simulink model "pid_active_suspension"  (R2024b)
settings: Solver=FixedStepAuto  StartTime=0.0  StopTime=10.0  FixedStep=0.001  MaxStep=0.001  RelTol=1e-3
undefined symbols (not defined in the file): A, B, C, D, kw, sigbuilder_block, T
libraries: slpidlib x1, simulink x1, dspfdesign x1
settings Model: Creator=11508  LastModifiedBy=11508
settings DataIOCC: SaveFormat=Array  ReturnWorkspaceOutputs=off
settings OptimizationCC: ReuseModelBlockBuffer=off
settings DebuggingCC: AlgebraicLoopMsg=none
settings RTWCC: GPUComputeCapability=3.5

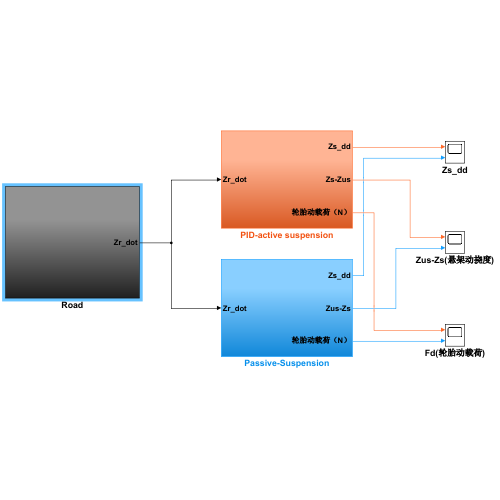
[thumbnail: Simulink's stored preview of the top-level diagram]
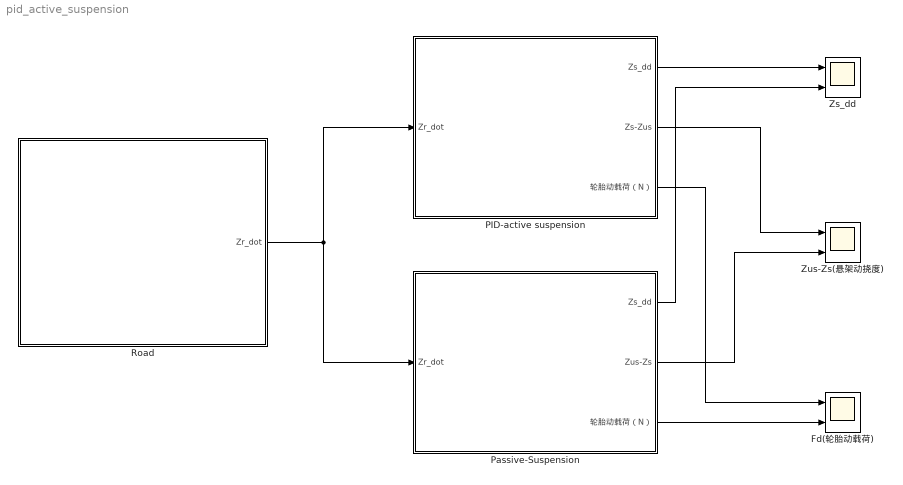
== system pid_active_suspension ==
  Fd(轮胎动载荷) : Scope  NumInputPorts=2
  PID-active suspension : Subsystem
  Passive-Suspension : Subsystem
  Road : Subsystem
  Zs_dd : Scope  NumInputPorts=2
  Zus-Zs(悬架动挠度) : Scope  NumInputPorts=2
  wires:
  PID-active suspension/1(Zs_dd) -> Zs_dd/1
  Passive-Suspension/1(Zs_dd) -> Zs_dd/2
  PID-active suspension/2(Zs-Zus) -> Zus-Zs(悬架动挠度)/1
  Passive-Suspension/2(Zus-Zs) -> Zus-Zs(悬架动挠度)/2
  Passive-Suspension/3(轮胎动载荷（N）) -> Fd(轮胎动载荷)/2
  PID-active suspension/3(轮胎动载荷（N）) -> Fd(轮胎动载荷)/1
  Road/1(Zr_dot) -> PID-active suspension/1(Zr_dot), Passive-Suspension/1(Zr_dot)

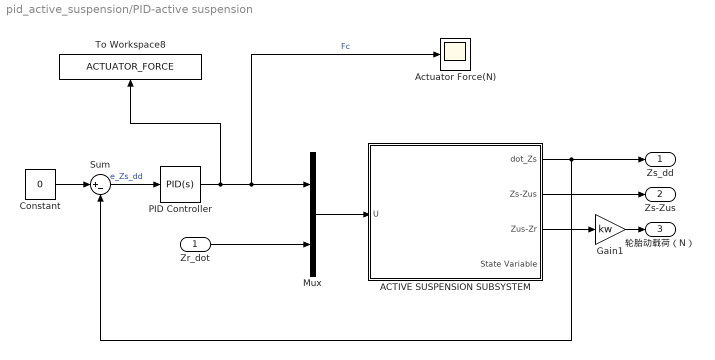
== system pid_active_suspension/PID-active suspension ==
  Zr_dot : Inport
  ACTIVE SUSPENSION SUBSYSTEM : Subsystem
  Actuator Force(N) : Scope
  Constant : Constant  Value=0
  Gain1 : Gain  Gain=kw
  Mux : Mux  Inputs=2
  PID Controller : slpidlib/PID Controller  Controller=PID  Form=Parallel  TimeDomain=Continuous-time  UseExternalTs=off  SampleTime=-1  IntegratorMethod=Forward Euler  FilterMethod=Forward Euler  ControllerParametersSource=internal  P=500  I=25  UseKiTs=off  D=10  UseExternalDerivativeSource=off  N=100  UseFilter=on  TunerSelectOption=Transfer Function Based (PID Tuner App)  InitialConditionSource=internal  InitialConditionForIntegrator=0  InitialConditionForFilter=0  DifferentiatorICPrevScaledInput=0  ExternalReset=none  TrackingMode=off  Kt=1  LimitOutput=off  SatLimitsSource=internal  UpperSaturationLimit=inf  LowerSaturationLimit=-inf  LinearizeAsGain=on  AntiWindupMode=none  Kb=1  LimitIntegrator=off  UpperIntegratorSaturationLimit=inf  LowerIntegratorSaturationLimit=-inf  POutMin=[]  POutMax=[]  IOutMin=[]  IOutMax=[]  DOutMin=[]  DOutMax=[]  NOutMin=[]  NOutMax=[]  SumOutMin=[]  SumOutMax=[]  SaturationOutMin=[]  SaturationOutMax=[]  PParamMin=[]  PParamMax=[]  IParamMin=[]  IParamMax=[]  DParamMin=[]  DParamMax=[]  NParamMin=[]  NParamMax=[]  KbParamMin=[]  KbParamMax=[]  KtParamMin=[]  KtParamMax=[]  KbOutMin=[]  KbOutMax=[]  KtOutMin=[]  KtOutMax=[]  IntegratorOutMin=[]  IntegratorOutMax=[]  FilterOutMin=[]  FilterOutMax=[]  SumI1OutMin=[]  SumI1OutMax=[]  SumI2OutMin=[]  SumI2OutMax=[]  SumI3OutMin=[]  SumI3OutMax=[]  SumI4OutMin=[]  SumI4OutMax=[]  SumDOutMin=[]  SumDOutMax=[]  DifferentiatorOutMin=[]  DifferentiatorOutMax=[]  FilterDiffOutCoefMin=[]  FilterDiffOutCoefMax=[]  ReciprocalOutMin=[]  ReciprocalOutMax=[]  SumDenOutMin=[]  SumDenOutMax=[]  SumNumOutMin=[]  SumNumOutMax=[]  DivideOutMin=[]  DivideOutMax=[]  UdiffTsProdOutMin=[]  UdiffTsProdOutMax=[]  NTsProdOutMin=[]  NTsProdOutMax=[]  UintegralTsProdOutMin=[]  UintegralTsProdOutMax=[]  UngainTsProdOutMin=[]  UngainTsProdOutMax=[]  ClampingZeroOutDataTypeStr=Inherit: Inherit via back propagation  ClampingZeroOutMin=[]  ClampingZeroOutMax=[]  FilterDenConstantOutDataTypeStr=Inherit: Inherit via back propagation  FilterDenConstantOutMin=[]  FilterDenConstantOutMax=[]  PCopyOutDataTypeStr=Inherit: Inherit via back propagation  PCopyOutMin=[]  PCopyOutMax=[]  NCopyOutDataTypeStr=Inherit: Inherit via back propagation  NCopyOutMin=[]  NCopyOutMax=[]  IntegratorContinuousStateAttributes=''  IntegratorStateMustResolveToSignalObject=off  IntegratorRTWStateStorageClass=Auto  FilterContinuousStateAttributes=''  FilterStateMustResolveToSignalObject=off  FilterRTWStateStorageClass=Auto  ParallelPVariant=InternalParameters  IdealPVariant=Disabled  IVariant=InternalParameters  DVariant=InternalParameters  IntegratorVariant=Continuous  SatVariant=Disabled  AWVariant=Passthrough  PCopyVariant=Disabled  TRVariant=Disabled  FdbkBlocksVariant=Forward  IdealPFdbkVariant=Disabled  SatFdbkVariant=Disabled  DerivativeFilterVariant=ContFilter  NVariant=InternalParameters  NCopyVariant=Disabled  FilterICVariant=InternalICsFilter  IntegratorICVariant=InternalICs  ExternalResetVariant=Disabled  TRSumVariant=Passthrough  SumFdbkVariant=Disabled  SumVariant=Sum_PID  TsampFilterVariant=InternalTs  TsampNgainVariant=Passthrough  TsampIntegralVariant=Disabled_SignalSpec  ExternalSaturationOutDataTypeStr=Inherit: Same as second input  DerivativeSourceVariant=ErrorSignal  PreIntVariant=InternalPreInt
  Sum : Sum  Inputs=|+-
  To Workspace8 : ToWorkspace  VariableName=ACTUATOR_FORCE  SampleTime=-1
  Zs_dd : Outport
  Zs-Zus : Outport  Port=2
  轮胎动载荷（N） : Outport  Port=3
  wires:
  Mux/1 -> ACTIVE SUSPENSION SUBSYSTEM/1(U)
  PID Controller/1 -> Mux/1, Actuator Force(N)/1, To Workspace8/1  "Fc"
  ACTIVE SUSPENSION SUBSYSTEM/2(Zs-Zus) -> Zs-Zus/1
  ACTIVE SUSPENSION SUBSYSTEM/3(Zus-Zr) -> Gain1/1
  Gain1/1 -> 轮胎动载荷（N）/1
  ACTIVE SUSPENSION SUBSYSTEM/1(dot_Zs) -> Sum/2, Zs_dd/1
  Zr_dot/1 -> Mux/2
  Constant/1 -> Sum/1
  Sum/1 -> PID Controller/1  "e_Zs_dd"

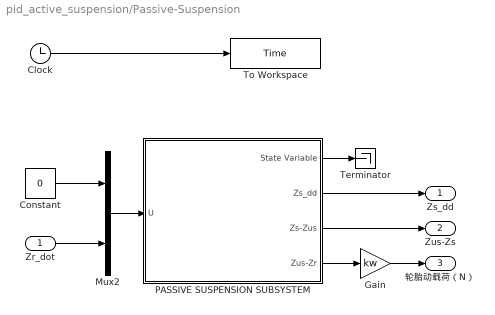
== system pid_active_suspension/Passive-Suspension ==
  Zr_dot : Inport
  Clock : Clock
  Constant : Constant  Value=0
  Gain : Gain  Gain=kw
  Mux2 : Mux  Inputs=2
  PASSIVE SUSPENSION SUBSYSTEM : Subsystem
  Terminator : Terminator
  To Workspace : ToWorkspace  VariableName=Time  SampleTime=-1
  Zs_dd : Outport
  Zus-Zs : Outport  Port=2
  轮胎动载荷（N） : Outport  Port=3
  wires:
  Mux2/1 -> PASSIVE SUSPENSION SUBSYSTEM/1(U)
  PASSIVE SUSPENSION SUBSYSTEM/3(Zs-Zus) -> Zus-Zs/1
  PASSIVE SUSPENSION SUBSYSTEM/2(Zs_dd) -> Zs_dd/1
  Gain/1 -> 轮胎动载荷（N）/1
  PASSIVE SUSPENSION SUBSYSTEM/4(Zus-Zr) -> Gain/1
  Zr_dot/1 -> Mux2/2
  Constant/1 -> Mux2/1
  Clock/1 -> To Workspace/1
  PASSIVE SUSPENSION SUBSYSTEM/1(State Variable) -> Terminator/1

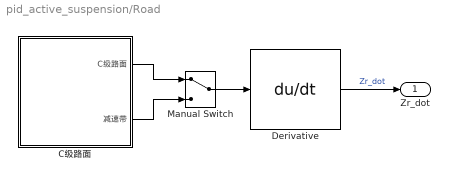
== system pid_active_suspension/Road ==
  C级路面 : Subsystem
  Derivative : Derivative
  Manual Switch : ManualSwitch
  Zr_dot : Outport
  wires:
  Derivative/1 -> Zr_dot/1  "Zr_dot"
  C级路面/2(减速带) -> Manual Switch/2
  C级路面/1(C级路面) -> Manual Switch/1
  Manual Switch/1 -> Derivative/1

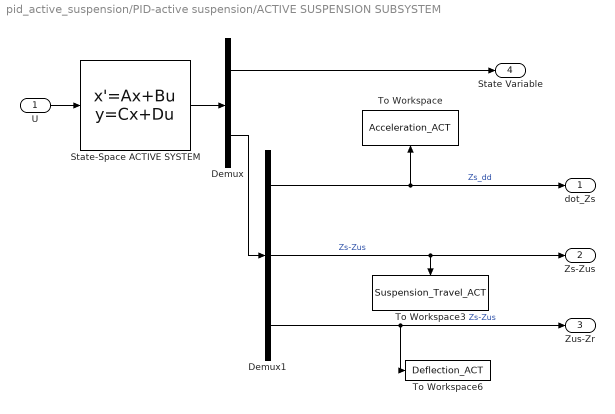
== system pid_active_suspension/PID-active suspension/ACTIVE SUSPENSION SUBSYSTEM ==
  U : Inport
  Demux : Demux  Outputs=[4 3]
  Demux1 : Demux  Outputs=3
  State-Space ACTIVE SYSTEM : StateSpace  A=A  B=cat(2,B,E)  C=cat(1,eye(4), C)  D=cat(1,zeros(4,2),cat(2,D,T))  InitialCondition=0
  To Workspace : ToWorkspace  VariableName=Acceleration_ACT  SampleTime=-1
  To Workspace3 : ToWorkspace  VariableName=Suspension_Travel_ACT  SampleTime=-1
  To Workspace6 : ToWorkspace  VariableName=Deflection_ACT  SampleTime=-1
  dot_Zs : Outport
  Zs-Zus : Outport  Port=2
  Zus-Zr : Outport  Port=3
  State Variable : Outport  Port=4
  wires:
  Demux/1 -> State Variable/1
  State-Space ACTIVE SYSTEM/1 -> Demux/1
  Demux1/1 -> To Workspace/1, dot_Zs/1  "Zs_dd"
  Demux1/2 -> To Workspace3/1, Zs-Zus/1  "Zs-Zus"
  U/1 -> State-Space ACTIVE SYSTEM/1
  Demux1/3 -> To Workspace6/1, Zus-Zr/1  "Zs-Zus"
  Demux/2 -> Demux1/1

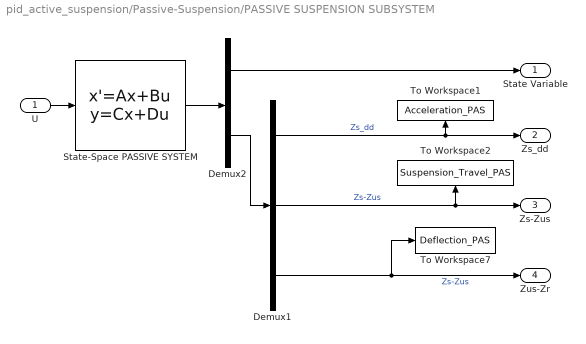
== system pid_active_suspension/Passive-Suspension/PASSIVE SUSPENSION SUBSYSTEM ==
  U : Inport
  Demux1 : Demux  Outputs=3
  Demux2 : Demux  Outputs=[4 3]
  State-Space PASSIVE SYSTEM : StateSpace  A=A  B=cat(2,B,E)  C=cat(1,eye(4), C)  D=cat(1,zeros(4,2),cat(2,D,T))  InitialCondition=0
  To Workspace1 : ToWorkspace  VariableName=Acceleration_PAS  SampleTime=-1
  To Workspace2 : ToWorkspace  VariableName=Suspension_Travel_PAS  SampleTime=-1
  To Workspace7 : ToWorkspace  VariableName=Deflection_PAS  SampleTime=-1
  State Variable : Outport
  Zs_dd : Outport  Port=2
  Zs-Zus : Outport  Port=3
  Zus-Zr : Outport  Port=4
  wires:
  State-Space PASSIVE SYSTEM/1 -> Demux2/1
  U/1 -> State-Space PASSIVE SYSTEM/1
  Demux2/1 -> State Variable/1
  Demux2/2 -> Demux1/1
  Demux1/1 -> Zs_dd/1, To Workspace1/1  "Zs_dd"
  Demux1/2 -> Zs-Zus/1, To Workspace2/1  "Zs-Zus"
  Demux1/3 -> Zus-Zr/1, To Workspace7/1  "Zs-Zus"

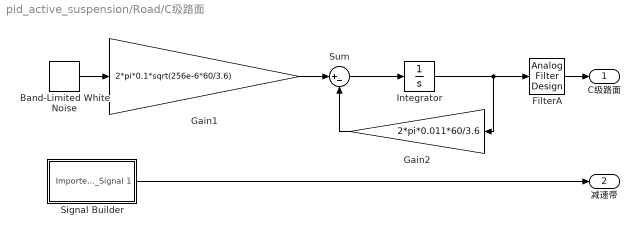
== system pid_active_suspension/Road/C级路面 ==
  Band-Limited White Noise : simulink/Sources/Band-Limited White Noise  Cov=0.5  Ts=0.01  seed=[23341]
  FilterA : dspfdesign/Analog Filter Design  method=Butterworth  filttype=Bandpass  N=4  Wlo=0.01*2*pi  Whi=20*2*pi  Rp=2  Rs=40
  Gain1 : Gain  Gain=2*pi*0.1*sqrt(256e-6*60/3.6)
  Gain2 : Gain  Gain=2*pi*0.011*60/3.6
  Integrator : Integrator
  Signal Builder : Subsystem  Tag=STV Subsys  LoadFcn=sigbuilder_block('load');  StartFcn=sigbuilder_block('start');  StopFcn=sigbuilder_block('stop');  ClipboardFcn=sigbuilder_block('clipboard');  mask(Sigbuilder block){tuvar=[0:10]}
      mask help: Simulink:masks:SigbuilderBlock_MD
      mask init:
      | if ~strcmp(get_param(bdroot(gcbh),'SimulationStatus'),'stopped') tuvar = sigbuilder_block('maskInit'); end
      settings: CopyFcn=sigbuilder_block('copy');  DeleteFcn=sigbuilder_block('delete');  ModelCloseFcn=sigbuilder_block('modelClose');  PreSaveFcn=sigbuilder_block('preSave');  PauseFcn=sigbuilder_block('pause');  ContinueFcn=sigbuilder_block('continue');  NameChangeFcn=sigbuilder_block('namechange');  OpenFcn=sigbuilder_block('open',[476.5 112.5 550.5 400 ]);  CloseFcn=sigbuilder_block('close');
      mask Display: plot(0, 0, 100, 100,[2, 2, 32, 32, 2], [68, 8, 8, 68, 68],[32, 2], [38, 38], [32, 19, 2],[53, 60, 44], [32, 17, 17, 2],[16, 16, 31, 31]);txt = getActiveGroup(gcbh);text(2, 100, txt,'verticalAlignment', 'top');
  Sum : Sum  Inputs=|+-
  C级路面 : Outport  VectorParamsAs1DForOutWhenUnconnected=off
  减速带 : Outport  Port=2  VectorParamsAs1DForOutWhenUnconnected=off
  wires:
  Signal Builder/1(Imported_Signal 1) -> 减速带/1
  Gain1/1 -> Sum/1
  Sum/1 -> Integrator/1
  Band-Limited White Noise/1 -> Gain1/1
  Integrator/1 -> Gain2/1, FilterA/1
  Gain2/1 -> Sum/2
  FilterA/1 -> C级路面/1

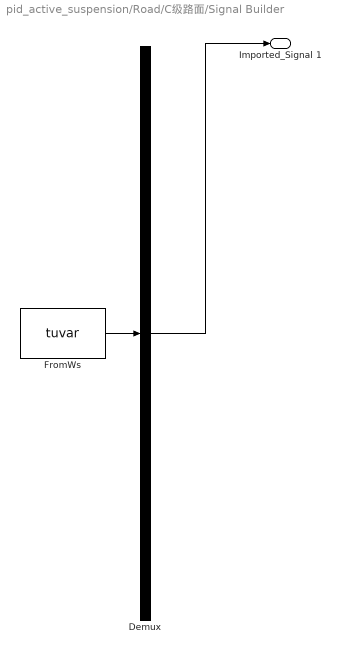
== system pid_active_suspension/Road/C级路面/Signal Builder ==
  Demux : Demux  Tag=STV Demux  Outputs=1
      settings: DisplayOption=none
  FromWs : FromWorkspace  Tag=STV FromWs  VariableName=tuvar
      SigBuilderData=|
      | common.afterFinalStr = 'Extrapolate'
      | common.sampleTime = 0
      | dataSet.timeRange = [0 4]
      | dataSet.name = 'Sheet1'
      | sbobj.Groups.Name = 'Sheet1'
      | sbobj.Groups.Signals.Name = 'Imported_Signal 1'
      | sbobj.Groups.Signals.XData = [0 0.001 0.002 0.003 0.004 0.005 0.006 0.007 0.008 0.009 0.01 0.011 ... (4001 elements, 1x4001)]
      | sbobj.Groups.Signals.YData = [0 0 0 0 0 0 0 0 0 0 0 0 ... (4001 elements, 1x4001)]
      | sbobj.Groups.TimeRange = [0 4]
  Imported_Signal 1 : Outport  Tag=STV Outport  VectorParamsAs1DForOutWhenUnconnected=off
  wires:
  Demux/1 -> Imported_Signal 1/1
  FromWs/1 -> Demux/1
